simulink model "Model"  (R2021b)
settings: Solver=VariableStepAuto  StartTime=0.0  StopTime=5  RelTol=1e-3
values from neighbouring files (symbols this model uses):
  A = [0 1;0 0]    [Calculation.m]
  b = [0;1]    [Calculation.m]
settings Model: Creator=16970  LastModifiedBy=16970

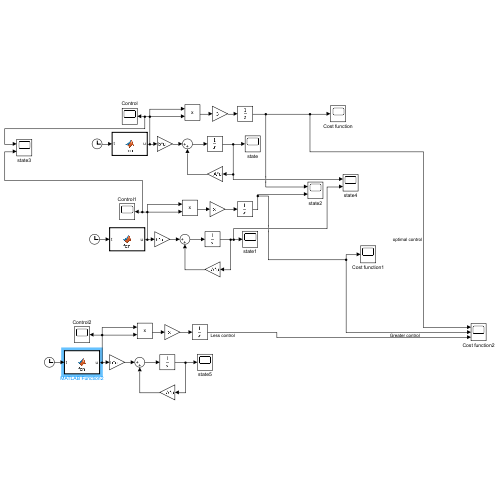
[thumbnail: Simulink's stored preview of the top-level diagram]
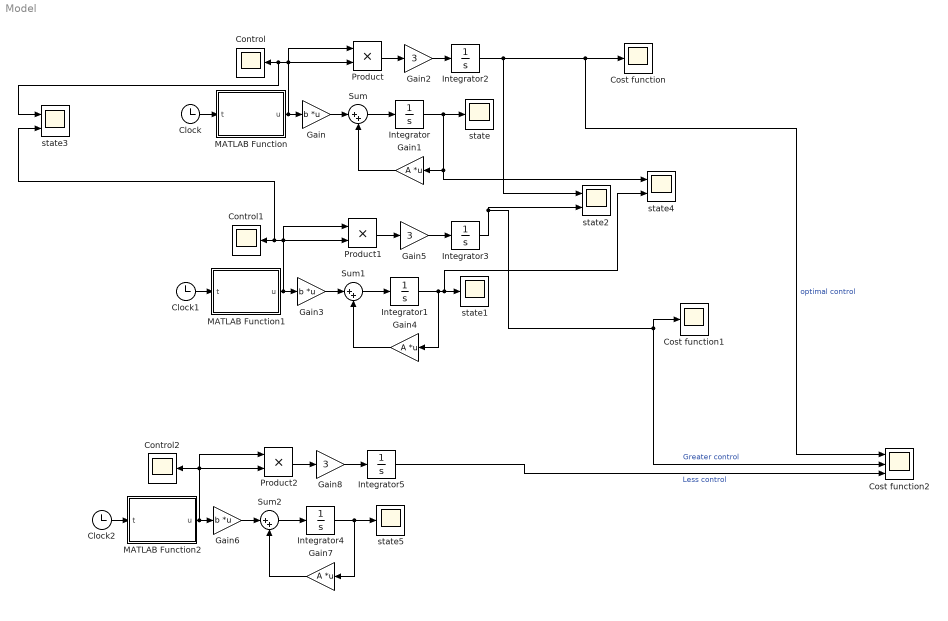
== system Model ==
  Clock : Clock
  Clock1 : Clock
  Clock2 : Clock
  Control : Scope
  Control1 : Scope
  Control2 : Scope
  Cost function : Scope
  Cost function1 : Scope
  Cost function2 : Scope  NumInputPorts=3
  Gain : Gain  Gain=b  Multiplication=Matrix(K*u)
  Gain1 : Gain  Gain=A  Multiplication=Matrix(K*u)
  Gain2 : Gain  Gain=3
  Gain3 : Gain  Gain=b  Multiplication=Matrix(K*u)
  Gain4 : Gain  Gain=A  Multiplication=Matrix(K*u)
  Gain5 : Gain  Gain=3
  Gain6 : Gain  Gain=b  Multiplication=Matrix(K*u)
  Gain7 : Gain  Gain=A  Multiplication=Matrix(K*u)
  Gain8 : Gain  Gain=3
  Integrator{,1..5} (6 alike) : Integrator
  MATLAB Function : MATLAB Function  TreatAsAtomicUnit=on
  MATLAB Function1 : MATLAB Function  TreatAsAtomicUnit=on
  MATLAB Function2 : MATLAB Function  TreatAsAtomicUnit=on
  Product : Product
  Product1 : Product
  Product2 : Product
  Sum : Sum  Inputs=|++
  Sum1 : Sum  Inputs=|++
  Sum2 : Sum  Inputs=|++
  state : Scope
  state1 : Scope
  state2 : Scope  NumInputPorts=2
  state3 : Scope  NumInputPorts=2
  state4 : Scope  NumInputPorts=2
  state5 : Scope
  wires:
  Clock/1 -> MATLAB Function/1(t)
  MATLAB Function/1(u) -> state3/1, Control/1, Product/1, Product/2, Gain/1
  Gain/1 -> Sum/1
  Sum/1 -> Integrator/1
  Gain1/1 -> Sum/2
  Integrator/1 -> state4/1, Gain1/1, state/1
  Product/1 -> Gain2/1
  Gain2/1 -> Integrator2/1
  Product1/1 -> Gain5/1
  Sum1/1 -> Integrator1/1
  MATLAB Function1/1(u) -> state3/2, Control1/1, Product1/1, Product1/2, Gain3/1
  Clock1/1 -> MATLAB Function1/1(t)
  Gain3/1 -> Sum1/1
  Gain4/1 -> Sum1/2
  Integrator1/1 -> state4/2, state1/1, Gain4/1
  Integrator2/1 -> state2/1, Cost function2/1, Cost function/1  "optimal control"
  Gain5/1 -> Integrator3/1
  Integrator3/1 -> state2/2, Cost function2/2, Cost function1/1  "Greater control"
  Gain8/1 -> Integrator5/1
  MATLAB Function2/1(u) -> Control2/1, Product2/1, Product2/2, Gain6/1
  Integrator4/1 -> state5/1, Gain7/1
  Gain7/1 -> Sum2/2
  Gain6/1 -> Sum2/1
  Sum2/1 -> Integrator4/1
  Clock2/1 -> MATLAB Function2/1(t)
  Product2/1 -> Gain8/1
  Integrator5/1 -> Cost function2/3  "Less control"

== matlab function Model/MATLAB Function ==
  data: t input; u output
function u = fcn(t)

u = 6/25 - (12*t)/125;

== matlab function Model/MATLAB Function2 ==
  data: t input; u output
function u = fcn(t)

u = 6/30 - (12*t)/130;

== matlab function Model/MATLAB Function1 ==
  data: t input; u output
function u = fcn(t)

u = 6/20 - (12*t)/120;
